simulink library "wrapToPi_ul"  (R2020a)
settings: Solver=VariableStepAuto  StartTime=0.0  StopTime=10.0  RelTol=1e-3
settings Model: Creator=Ayaz  LastModifiedBy=Ayaz

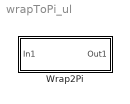
== system wrapToPi_ul ==
  Wrap2Pi : Subsystem
      mask Display: disp('Wrap to Pi')

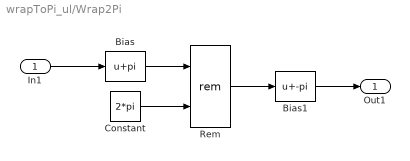
== system wrapToPi_ul/Wrap2Pi ==
  In1 : Inport
  Bias : Bias  Bias=pi
  Bias1 : Bias  Bias=-pi
  Constant : Constant  Value=2*pi
  Rem : Math  Operator=rem  SaturateOnIntegerOverflow=on
  Out1 : Outport
  wires:
  In1/1 -> Bias/1
  Constant/1 -> Rem/2
  Bias/1 -> Rem/1
  Rem/1 -> Bias1/1
  Bias1/1 -> Out1/1
